simulink model "robot"  (R2018a)
settings: Solver=VariableStepAuto  StartTime=0.0  StopTime=10.0  RelTol=1e-3
values from neighbouring files (symbols this model uses):
  K_theta = 3    [robot_input.m]
  Kv = 4    [robot_input.m]
  L = 10    [robot_input.m]
  X_zv = 10    [robot_input.m]
  Y_zv = 80    [robot_input.m]
libraries: simulink x1
settings Model: Creator=zises  LastModifiedBy=User

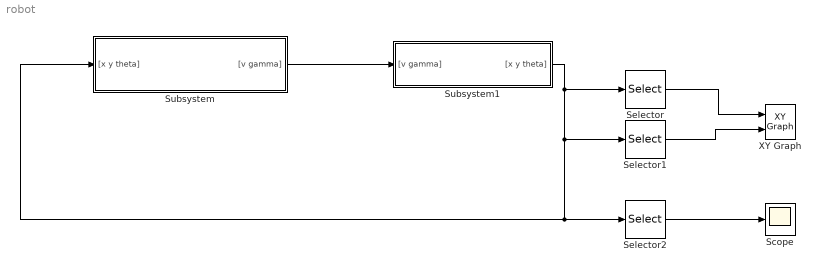
== system robot ==
  Scope : Scope
  Selector : Selector  InputPortWidth=3  IndexOptions=Index vector (dialog)  Indices=1  OutputSizes=1
  Selector1 : Selector  InputPortWidth=3  IndexOptions=Index vector (dialog)  Indices=2  OutputSizes=1
  Selector2 : Selector  InputPortWidth=3  IndexOptions=Index vector (dialog)  Indices=[1 2]  OutputSizes=1
  Subsystem : Subsystem
  Subsystem1 : Subsystem
  XY Graph : simulink/Sinks/XY Graph  xmin=0  xmax=100  ymin=0  ymax=100  st=-1
  wires:
  Subsystem/1("[v gamma]") -> Subsystem1/1("[v gamma]")
  Subsystem1/1("[x y theta]") -> Subsystem/1("[x y theta]"), Selector2/1, Selector1/1, Selector/1
  Selector/1 -> XY Graph/1
  Selector1/1 -> XY Graph/2
  Selector2/1 -> Scope/1

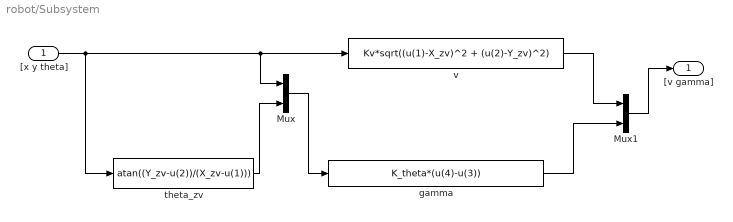
== system robot/Subsystem ==
  "[x y theta]" : Inport
  Mux : Mux  Inputs=2
  Mux1 : Mux  Inputs=2
  gamma : Fcn  Expr=K_theta*(u(4)-u(3))
  theta_zv : Fcn  Expr=atan((Y_zv-u(2))/(X_zv-u(1)))
  v : Fcn  Expr=Kv*sqrt((u(1)-X_zv)^2 + (u(2)-Y_zv)^2)
  "[v gamma]" : Outport
  wires:
  theta_zv/1 -> Mux/2
  "[x y theta]"/1 -> v/1, Mux/1, theta_zv/1
  Mux/1 -> gamma/1
  v/1 -> Mux1/1
  gamma/1 -> Mux1/2
  Mux1/1 -> "[v gamma]"/1

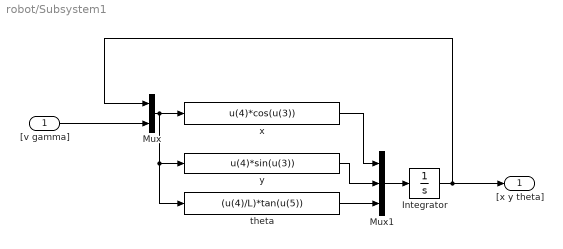
== system robot/Subsystem1 ==
  "[v gamma]" : Inport
  Integrator : Integrator
  Mux : Mux  Inputs=2
  Mux1 : Mux  Inputs=3
  theta : Fcn  Expr=(u(4)/L)*tan(u(5))
  x : Fcn  Expr=u(4)*cos(u(3))
  y : Fcn  Expr=u(4)*sin(u(3))
  "[x y theta]" : Outport
  wires:
  y/1 -> Mux1/2
  Integrator/1 -> Mux/1, "[x y theta]"/1
  theta/1 -> Mux1/3
  Mux1/1 -> Integrator/1
  "[v gamma]"/1 -> Mux/2
  x/1 -> Mux1/1
  Mux/1 -> theta/1, y/1, x/1
